simulink model "CommSysSimulink_Project2"  (R2024b)
settings: Solver=VariableStepAuto  StartTime=0.0  StopTime=inf  RelTol=1e-3
model workspace (MAT data in the model file):
  Data_Aided_Synchronisation = Simulink.Parameter
  Data_Aided_Synchronisation.Value = 0
  Data_Aided_Synchronisation.Complexity = 'real'
  Data_Aided_Synchronisation.Dimensions = [1 1]
  Data_Aided_Synchronisation.DataType = 'auto'
  Frequency_Locked_Loop = Simulink.Parameter
  Frequency_Locked_Loop.Value = 0
  Frequency_Locked_Loop.Complexity = 'real'
  Frequency_Locked_Loop.Dimensions = [1 1]
  Frequency_Locked_Loop.DataType = 'auto'
  Phase_Locked_Loop = Simulink.Parameter
  Phase_Locked_Loop.Value = 0
  Phase_Locked_Loop.Complexity = 'real'
  Phase_Locked_Loop.Dimensions = [1 1]
  Phase_Locked_Loop.DataType = 'auto'
  Symbol_Synchronisation = Simulink.Parameter
  Symbol_Synchronisation.Value = 0
  Symbol_Synchronisation.Complexity = 'real'
  Symbol_Synchronisation.Dimensions = [1 1]
  Symbol_Synchronisation.DataType = 'auto'
  Use_Costas_Loop = Simulink.Parameter
  Use_Costas_Loop.Value = 0
  Use_Costas_Loop.Complexity = 'real'
  Use_Costas_Loop.Dimensions = [1 1]
  Use_Costas_Loop.DataType = 'auto'
  iSNR = 1
  x = 0
undefined symbols (not defined in the file): alpha, fCRes, filterLenSymbols, modOrder, phaseOffsets, phaseOffsetSelector, samplesPerSymbol, SNR, symRate
libraries: commdigbbndpm3 x6, commsync2 x5, commrfcorlib x3, simulink x2, commfilt2 x2, commdigbbndam3 x2, commchan3 x1, commsink2 x1, commseqgen3 x1, commrandsrc3 x1, commrflib2 x1
settings Model: Creator=flora  LastModifiedBy=Sukhman

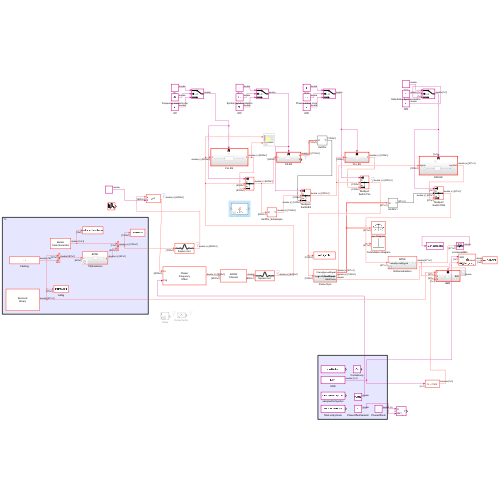
[thumbnail: Simulink's stored preview of the top-level diagram]
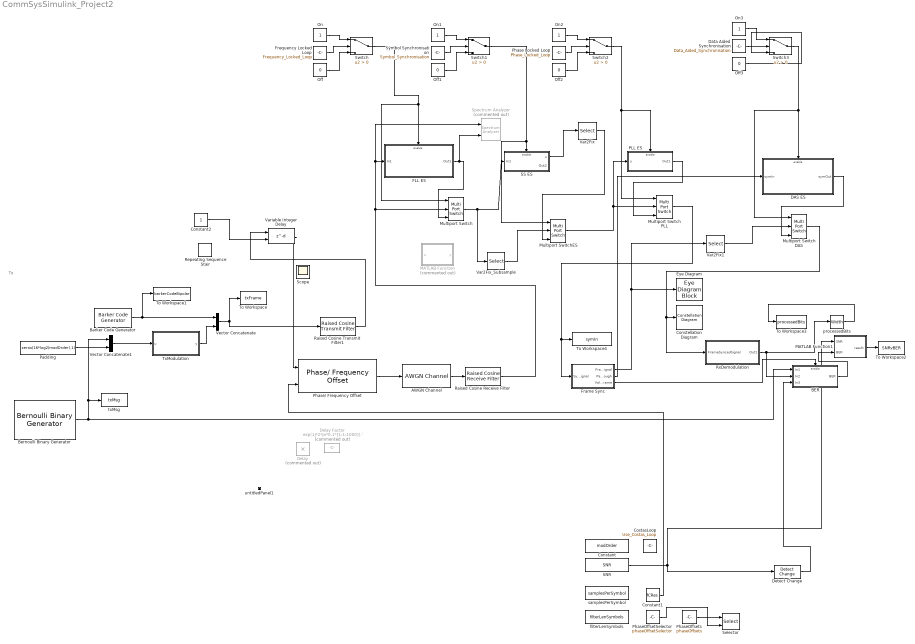
== system CommSysSimulink_Project2 ==
  note: Tx
  AWGN Channel : commchan3/AWGN Channel  LegacyMode=off  NoiseMethod="Signal to noise ratio  (Eb/No)"  noiseMode="Signal to noise ratio  (SNR)"  EbNo=SNR  EsNo=10  SNR=SNR  BitsPerSymbol=log2(modOrder)  SignalPower=1/samplesPerSymbol  SamplesPerSymbol=samplesPerSymbol  SymbolPeriod=1  VarianceSource=Parameter  Variance=SNR/2  RandomStream=Global stream  Seed=67  SimulateUsing=Interpreted execution
  BER : Subsystem  TreatAsAtomicUnit=on
  Barker Code Generator : commseqgen3/Barker Code Generator  Length=7  LengthSimulink=13  SampleTime=-1  SamplesPerFrame=13  OutputDataType=double  SimulateUsing=Interpreted execution
  Bernoulli Binary Generator : commrandsrc3/Bernoulli Binary Generator  ProbabilityOfZero=0.5  SeedSource=Auto  Seed=0  SampleTime=1/(symRate*log2(modOrder))  SamplesPerFrame="(symRate  - 13 -16) * log2(modOrder)"  OutputDataType=double  SimulateUsing=Interpreted execution
  Constant : Constant  Value=modOrder
  Constant1 : Constant  Value=fCRes
  Constant2 : Constant
  Constellation Diagram : ConstellationDiagram  WindowPosition=[527.000000,241.000000,653.000000,585.000000,]  Visible=on  ScopeFrameLocation=window  ReferenceConstellation=BPSK  XLimits=[-1.375,1.375]  YLimits=[-1.375,1.375]  MaximizeAxes=on
  CostasLoop : Constant  Value=Use_Costas_Loop
  DAS ES : Subsystem  TreatAsAtomicUnit=on
  Data Aided Synchronisation : Constant  Value=Data_Aided_Synchronisation  VectorParams1D=off
  Delay : Product  Commented=on  LockScale=on
  Delay Factor : Constant  Commented=on  Value=exp(1j*2*pi*0.1*[1:1:1000]).'  VectorParams1D=off  SampleTime=0.971  LockScale=on
  Detect Change : simulink/Logic and Bit Operations/Detect Change  vinit=0  OutDataTypeStr=boolean
  Eye Diagram : EyeDiagramBlock  WindowPosition=[302.000000,4.000000,1167.000000,855.000000,]  Visible=on  ScopeFrameLocation=window
  FLL ES : Subsystem  TreatAsAtomicUnit=on
  Frame Sync : Subsystem
  Frequency Locked Loop : Constant  Value=Frequency_Locked_Loop
  MATLAB Function : MATLAB Function  Commented=on  TreatAsAtomicUnit=on
  MATLAB Function1 : MATLAB Function  TreatAsAtomicUnit=on
  Multiport Switch : MultiPortSwitch  DataPortOrder=Zero-based contiguous  Inputs=2  zeroidx=on  SaturateOnIntegerOverflow=off  InputSameDT=off
  Multiport Switch DAS : MultiPortSwitch  DataPortOrder=Zero-based contiguous  Inputs=2  zeroidx=on  SaturateOnIntegerOverflow=off  InputSameDT=off
  Multiport Switch PLL : MultiPortSwitch  DataPortOrder=Zero-based contiguous  Inputs=2  zeroidx=on  SaturateOnIntegerOverflow=off  InputSameDT=off
  Multiport SwitchES : MultiPortSwitch  DataPortOrder=Zero-based contiguous  Inputs=2  zeroidx=on  SaturateOnIntegerOverflow=off  InputSameDT=off
  Off{,1..3} (4 alike) : Constant  Value=0
  On{,1..3} (4 alike) : Constant
  PLL ES : Subsystem  TreatAsAtomicUnit=on
  Padding : Constant  Value=zeros(16*log2(modOrder),1)  SampleTime=-1
  Phase Locked Loop : Constant  Value=Phase_Locked_Loop
  Phase/ Frequency Offset : commrflib2/Phase// Frequency Offset  phaseOffset=rad2deg(phaseOffsets(phaseOffsetSelector))  freqPort=on  freqOffset=100
      settings: LibrarySourceBlock=|
      | commrfcorlib/Phase//
      | Frequency
      | Offset
  PhaseOffsetSelector : Constant  Value=phaseOffsetSelector
  PhaseOffsets : Constant  Value=phaseOffsets
  Raised Cosine Receive Filter : commfilt2/Raised Cosine Receive Filter  filtType=Square root  R=alpha  filtSpan=filterLenSymbols  N=samplesPerSymbol  downFactor=1  downOffset=0  filterGain=1  InputProcessing=Columns as channels (frame based)  RateOptions=Enforce single-rate processing  framing=Mute  checkCoeff=on  variableName=rcRxFilt  currentFiltSpan=10  D=5  inputOffset=0  sampMode=Mute  saveAsFlag=0  rateMode=Downsampling  checkGain=Normalized  launchFVT=on  roundingMode=Floor  overflowMode=off  coeffDataTypeStr=Inherit: Same word length as input  coeffMin=[]  coeffMax=[]  coeffLastDataTypeStr=Inherit: Same word length as input  accumDataTypeStr=Inherit: Same as product output  accumLastDataTypeStr=Inherit: Same as product output  outputDataTypeStr=Inherit: Same as accumulator  outputMin=[]  outputMax=[]  outputLastDataTypeStr=Inherit: Same as accumulator
  Raised Cosine Transmit Filter1 : commfilt2/Raised Cosine Transmit Filter  filtType=Square root  R=alpha  filtSpan=filterLenSymbols  N=samplesPerSymbol  filterGain=1  InputProcessing=Columns as channels (frame based)  RateOptions=Enforce single-rate processing  framing=Mute  checkCoeff=on  variableName=rcTxFilt  checkGain=Normalized  sampMode=Mute  saveAsFlag=0  currentFiltSpan=10  D=(10)/2  launchFVT=on  roundingMode=Floor  overflowMode=off  coeffDataTypeStr=Inherit: Same word length as input  coeffMin=[]  coeffMax=[]  coeffLastDataTypeStr=Inherit: Same word length as input  outputDataTypeStr=Inherit: Same as accumulator  outputMin=[]  outputMax=[]  outputLastDataTypeStr=Inherit: Same as accumulator
  Repeating Sequence Stair : simulink/Sources/Repeating Sequence Stair  OutValues=[3 1 4 2 1].'  tsamp=-1  OutMin=[]  OutMax=[]  OutDataTypeStr=double  OutputDataTypeScalingMode=double  OutDataType=fixdt(0,8)  ConRadixGroup=Best Precision: Vector-wise  OutScaling=2^-12
      settings: LibrarySourceBlock=|
      | hdlsllib/Sources/Repeating
      | Sequence
      | Stair
  RxDemodulation : Subsystem  Variant=on
  SNR : Constant  Value=SNR  VectorParams1D=off
  SS ES : Subsystem  TreatAsAtomicUnit=on
  Selector : Selector  InputPortWidth=5  IndexOptions=Index vector (port)  Indices=[1 3]  OutputSizes=1
  Spectrum Analyzer : SpectrumAnalyzer  Commented=on  NumInputPorts=2  WindowPosition=[-1976.000000,107.000000,1455.000000,953.000000,]  Visible=on  ScopeFrameLocation=window  ViewType=Spectrum and spectrogram  PlotAsTwoSidedSpectrum=off  Span=399999.99999999994  StartFrequency=-199999.99999999997  StopFrequency=199999.99999999997  YLimits=[-112.84937781743083,24.09936467256917]  ColorLimits=[-112.30807844,24.64066405]  ExpandToolstrip=on
  Switch{,1..3} (4 alike) : Switch  Criteria=u2 > Threshold  SaturateOnIntegerOverflow=off  InputSameDT=off
  Symbol Synchronisation : Constant  Value=Symbol_Synchronisation
  To Workspace : ToWorkspace  VariableName=txFrame  SampleTime=-1
      settings: Save2DSignal=2-D array (concatenate along first dimension)
  To Workspace1 : ToWorkspace  VariableName=barkerCodeBipolar  SampleTime=-1
      settings: Save2DSignal=2-D array (concatenate along first dimension)
  To Workspace2 : ToWorkspace  VariableName=SNRvBER  SampleTime=-1
  To Workspace3 : ToWorkspace  VariableName=processedBits  SaveFormat=Timeseries  SampleTime=-1
  To Workspace4 : ToWorkspace  VariableName=symIn  SampleTime=-1
  TxModulation : Subsystem  Variant=on
  Var2Fix : Selector  InputPortWidth=symRate*1.1  IndexOptions=Starting index (dialog)  Indices=1  OutputSizes=symRate
  Var2Fix1 : Selector  InputPortWidth=symRate-13-16  IndexOptions=Starting index (dialog)  Indices=1  OutputSizes=symRate-13-16
  Var2Fix_Subsample : Selector  InputPortWidth=symRate*samplesPerSymbol  IndexOptions=Index vector (dialog)  Indices=[1: samplesPerSymbol : symRate*samplesPerSymbol]  OutputSizes=symRate*samplesPerSymbol
  Variable Integer Delay : Delay  DelayLengthSource=Input port  InputProcessing=Columns as channels (frame based)
      settings: InputPortMap=u0,p1
  Vector Concatenate : Concatenate
  Vector Concatenate1 : Concatenate
  filterLenSymbols : Constant  Value=filterLenSymbols
  processedBits : Width
  samplesPerSymbol : Constant  Value=samplesPerSymbol
  txMsg : ToWorkspace  VariableName=txMsg  SampleTime=-1
      settings: Save2DSignal=2-D array (concatenate along first dimension)
  untitledPanel1 : Subsystem  Tag=HiddenForWebPanel  IsWebBlockPanel=on
  Scope : Scope
  wires:
  BER/1(BER) -> MATLAB Function1/2(BER)
  processedBits/1 -> To Workspace3/1
  Detect Change/1 -> BER/3(In3)
  Frame Sync/1(FrameSyncedSignal) -> Var2Fix1/1, Eye Diagram/1
  AWGN Channel/1 -> Raised Cosine Receive Filter/1
  MATLAB Function1/1(result) -> To Workspace2/1
  RxDemodulation/1(Out1) -> processedBits/1, BER/2(In2)
  SNR/1 -> MATLAB Function1/1(SNR), Detect Change/1
  Frame Sync/3(ValidFrame) -> BER/Enable
  Bernoulli Binary Generator/1 -> txMsg/1, Vector Concatenate1/1, BER/1(In1)
  Barker Code Generator/1 -> Vector Concatenate/1, To Workspace1/1
  Vector Concatenate1/1 -> TxModulation/1(u)
  TxModulation/1(y) -> Vector Concatenate/2
  Padding/1 -> Vector Concatenate1/2
  Vector Concatenate/1 -> To Workspace/1, Raised Cosine Transmit Filter1/1
  Phase/ Frequency Offset/1 -> AWGN Channel/1
  PhaseOffsets/1 -> Selector/1
  PhaseOffsetSelector/1 -> Selector/2
  Constant1/1 -> Phase/ Frequency Offset/2
  On/1 -> Switch/1
  Off/1 -> Switch/3
  Frequency Locked Loop/1 -> Switch/2
  Switch/1 -> Multiport Switch/1, FLL ES/Enable
  Symbol Synchronisation/1 -> Switch1/2
  On1/1 -> Switch1/1
  Off1/1 -> Switch1/3
  Phase Locked Loop/1 -> Switch2/2
  Off2/1 -> Switch2/3
  On2/1 -> Switch2/1
  Switch1/1 -> Multiport SwitchES/1, SS ES/Enable
  Raised Cosine Receive Filter/1 -> Spectrum Analyzer/1, FLL ES/1(In1), Multiport Switch/2
  FLL ES/1(Out1) -> Spectrum Analyzer/2, Multiport Switch/3
  Multiport Switch/1 -> SS ES/1(In1), Var2Fix_Subsample/1
  Switch2/1 -> Multiport Switch PLL/1, PLL ES/Enable
  SS ES/1(u) -> Var2Fix/1
  PLL ES/1(Out1) -> Multiport Switch PLL/3
  Multiport Switch PLL/1 -> Frame Sync/1(SymbolSyncedSignal), To Workspace4/1
  Var2Fix/1 -> Multiport SwitchES/3
  Multiport SwitchES/1 -> PLL ES/1(u), Multiport Switch PLL/2
  Var2Fix_Subsample/1 -> Multiport SwitchES/2
  Raised Cosine Transmit Filter1/1 -> Variable Integer Delay/1
  Off3/1 -> Switch3/3
  Data Aided Synchronisation/1 -> Switch3/2
  On3/1 -> Switch3/1
  Switch3/1 -> Multiport Switch DAS/1, DAS ES/Enable
  DAS ES/1(symOut) -> Multiport Switch DAS/3
  Frame Sync/2(Passthrough) -> DAS ES/1(symIn)
  Multiport Switch DAS/1 -> RxDemodulation/1(FrameSyncedSignal), Constellation Diagram/1
  Var2Fix1/1 -> Multiport Switch DAS/2
  Constant2/1 -> Variable Integer Delay/2
  Variable Integer Delay/1 -> Phase/ Frequency Offset/1

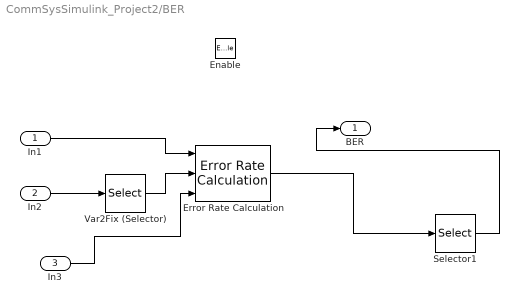
== system CommSysSimulink_Project2/BER ==
  In1 : Inport
  In2 : Inport  Port=2
  In3 : Inport  Port=3
  Enable : EnablePort  PropagateVarSize=During execution
  Error Rate Calculation : commsink2/Error Rate Calculation  N=0  st_delay=0  cp_mode=Entire frame  subframe=[]  PMode=Port  WsName=ErrorVec  RsMode2=on  stop=off  numErr=100  maxBits=1e6
      settings: LibrarySourceBlock=|
      | commhdlsink/Error Rate
      | Calculation
  Selector1 : Selector  InputPortWidth=3  IndexOptions=Index vector (dialog)  Indices=1  OutputSizes=1
  Var2Fix (Selector) : Selector  IndexOptions=Starting index (dialog)  Indices=1  OutputSizes="(symRate  - 13 -16) * log2(modOrder)"
  BER : Outport
  wires:
  In1/1 -> Error Rate Calculation/1
  Var2Fix (Selector)/1 -> Error Rate Calculation/2
  Error Rate Calculation/1 -> Selector1/1
  Selector1/1 -> BER/1
  In2/1 -> Var2Fix (Selector)/1
  In3/1 -> Error Rate Calculation/3

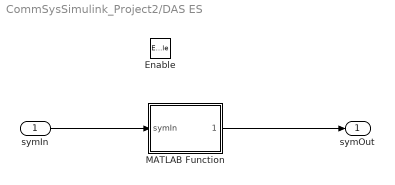
== system CommSysSimulink_Project2/DAS ES ==
  symIn : Inport
  Enable : EnablePort
  MATLAB Function : MATLAB Function  TreatAsAtomicUnit=on
  symOut : Outport
  wires:
  symIn/1 -> MATLAB Function/1(symIn)
  MATLAB Function/1(symOut) -> symOut/1

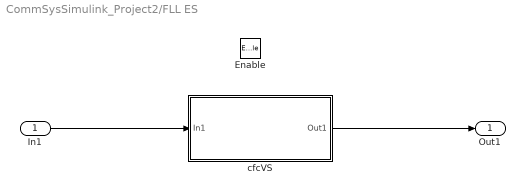
== system CommSysSimulink_Project2/FLL ES ==
  In1 : Inport
      settings: SignalType=complex
  Enable : EnablePort
  cfcVS : Subsystem  Variant=on
  Out1 : Outport
  wires:
  cfcVS/1(Out1) -> Out1/1
  In1/1 -> cfcVS/1(In1)

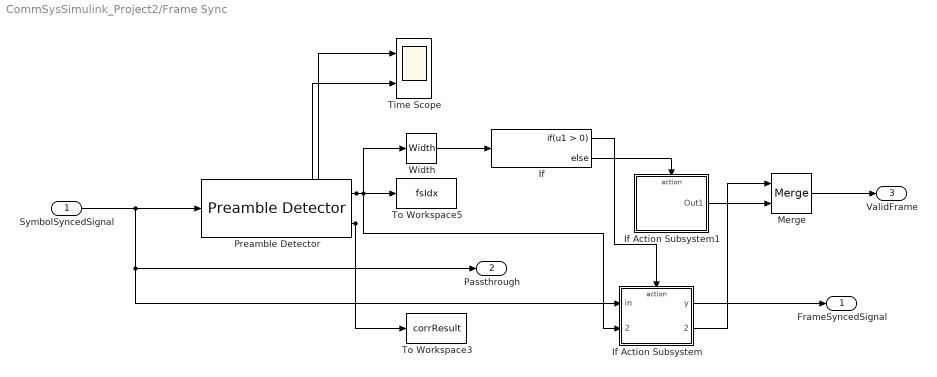
== system CommSysSimulink_Project2/Frame Sync ==
  SymbolSyncedSignal : Inport
  If : If
  If Action Subsystem : Subsystem  TreatAsAtomicUnit=on
  If Action Subsystem1 : Subsystem  TreatAsAtomicUnit=on
  Merge : Merge
  Preamble Detector : commsync2/Preamble Detector  Input=Symbol  Preamble=[-1;-1;-1;-1;-1;1;1;-1;-1;1;-1;1;-1]  Threshold=5  DetectionMetricOutput=on  Detections=First  SimulateUsing=Interpreted execution
  Time Scope : Scope  NumInputPorts=2
  To Workspace3 : ToWorkspace  VariableName=corrResult  SaveFormat=Timeseries  SampleTime=-1
      settings: Save2DSignal=2-D array (concatenate along first dimension)
  To Workspace5 : ToWorkspace  VariableName=fsIdx  SaveFormat=Structure  SampleTime=-1
  Width : Width
  FrameSyncedSignal : Outport
  Passthrough : Outport  Port=2
  ValidFrame : Outport  Port=3
  wires:
  If Action Subsystem/1(y) -> FrameSyncedSignal/1
  Merge/1 -> ValidFrame/1
  Width/1 -> If/1
  Preamble Detector/2 -> To Workspace3/1, Time Scope/2
  If/1 -> If Action Subsystem/Action
  Preamble Detector/1 -> Time Scope/1, If Action Subsystem/2(peakIdx), To Workspace5/1, Width/1
  If Action Subsystem1/1(Out1) -> Merge/2
  If/2 -> If Action Subsystem1/Action
  SymbolSyncedSignal/1 -> Preamble Detector/1, Passthrough/1, If Action Subsystem/1(in)
  If Action Subsystem/2(ValidFrame) -> Merge/1

== system CommSysSimulink_Project2/PLL ES ==
  u : Inport
  Enable : EnablePort  PropagateVarSize=During execution
  Variant Subsystem : Subsystem  Variant=on
  Out1 : Outport
  wires:
  u/1 -> Variant Subsystem/1(u)
  Variant Subsystem/1(y) -> Out1/1

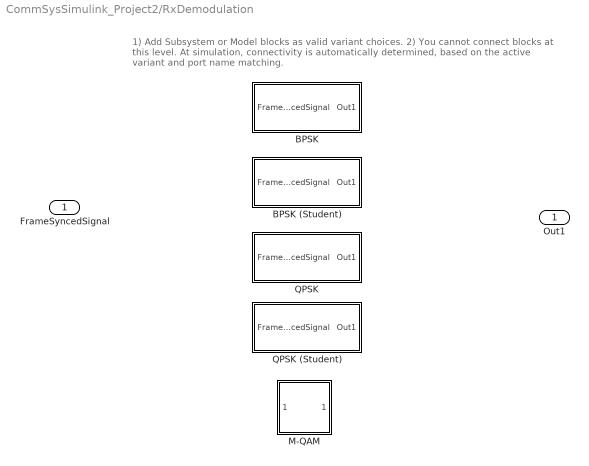
== system CommSysSimulink_Project2/RxDemodulation ==
  note: 1) Add Subsystem or Model blocks as valid variant choices.
      | 2) You cannot connect blocks at this level. At simulation, connectivity is automatically
      | determined, based on the active variant and port name matching.
  FrameSyncedSignal : Inport
  BPSK : Subsystem  VariantControl="modScheme==\"BPSK\""
  BPSK (Student) : Subsystem  VariantControl="modScheme==\"BPSK (Student)\""
  M-QAM : Subsystem  VariantControl="modScheme==\"M-QAM\""
  QPSK : Subsystem  VariantControl="modScheme==\"QPSK\""
  QPSK (Student) : Subsystem  VariantControl="modScheme==\"QPSK (Student)\""
  Out1 : Outport

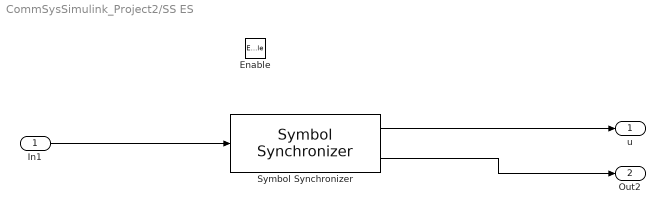
== system CommSysSimulink_Project2/SS ES ==
  In1 : Inport
  Enable : EnablePort  PropagateVarSize=During execution
  Symbol Synchronizer : commsync2/Symbol Synchronizer  Modulation=PAM/PSK/QAM  TimingErrorDetector=Zero-Crossing (decision-directed)  SamplesPerSymbol=samplesPerSymbol  DampingFactor=1  NormalizedLoopBandwidth=0.01  DetectorGain=2.7  TimingErrorOutputPort=on  SimulateUsing=Code generation
  u : Outport
      settings: SignalType=complex
  Out2 : Outport  Port=2
  wires:
  In1/1 -> Symbol Synchronizer/1
  Symbol Synchronizer/1 -> u/1
  Symbol Synchronizer/2 -> Out2/1

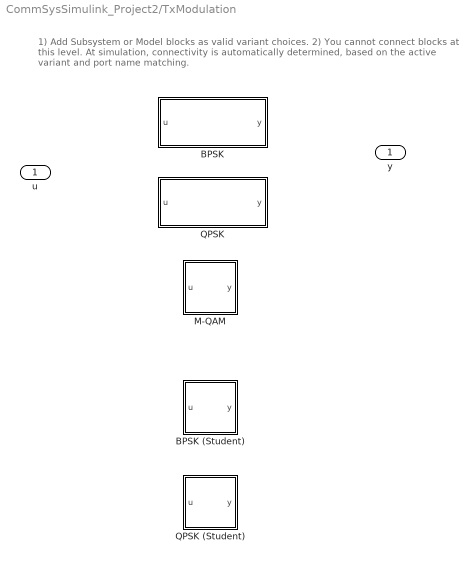
== system CommSysSimulink_Project2/TxModulation ==
  note: 1) Add Subsystem or Model blocks as valid variant choices.
      | 2) You cannot connect blocks at this level. At simulation, connectivity is automatically
      | determined, based on the active variant and port name matching.
  u : Inport
  BPSK : Subsystem  VariantControl="modScheme==\"BPSK\""
  BPSK (Student) : Subsystem  VariantControl="modScheme==\"BPSK (Student)\""
  M-QAM : Subsystem  VariantControl="modScheme==\"M-QAM\""
  QPSK : Subsystem  VariantControl="modScheme==\"QPSK\""
  QPSK (Student) : Subsystem  VariantControl="modScheme==\"QPSK (Student)\""
  y : Outport

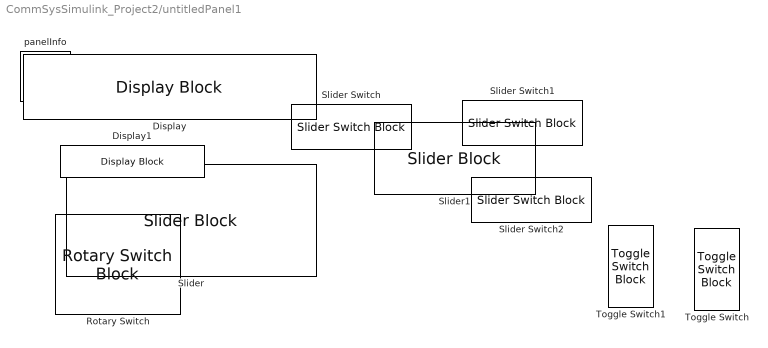
== system CommSysSimulink_Project2/untitledPanel1 ==
  Display : DisplayBlock  Tag=HiddenForWebPanel  PanelInfo="{\"height\":25,\"left\":685,\"panelId\":\"panelId-f31e1c61-8a53-45bb-afd0-f88e0f139d22\",\"top\":114,\"type\":\"panelChild\",\"version\":\"2019b\",\"width\":131,\"zIndex\":1500002}"  LabelPosition=Hide  Transparency=1
  Display1 : DisplayBlock  Tag=HiddenForWebPanel  PanelInfo="{\"height\":30,\"left\":680,\"panelId\":\"panelId-f31e1c61-8a53-45bb-afd0-f88e0f139d22\",\"top\":36,\"type\":\"panelChild\",\"version\":\"2019b\",\"width\":135,\"zIndex\":1500008}"  LabelPosition=Hide  Transparency=1
  Rotary Switch : RotarySwitchBlock  Tag=HiddenForWebPanel  PanelInfo="{\"height\":100,\"left\":271,\"panelId\":\"panelId-f31e1c61-8a53-45bb-afd0-f88e0f139d22\",\"top\":38,\"type\":\"panelChild\",\"version\":\"2019b\",\"width\":125,\"zIndex\":1500010}"  LabelPosition=Hide
      settings: Values={{'0', 'pi/8', 'pi/4', 'pi/2', 'pi'}, [1 2 3 4 5]}
  Slider : SliderBlock  Tag=HiddenForWebPanel  PanelInfo="{\"height\":88,\"left\":43,\"panelId\":\"panelId-f31e1c61-8a53-45bb-afd0-f88e0f139d22\",\"top\":53,\"type\":\"panelChild\",\"version\":\"2019b\",\"width\":191,\"zIndex\":1500006}"  ScaleMin=-30  ScaleMax=30
  Slider Switch : SliderSwitchBlock  Tag=HiddenForWebPanel  PanelInfo="{\"height\":45,\"left\":65,\"panelId\":\"panelId-f31e1c61-8a53-45bb-afd0-f88e0f139d22\",\"top\":226,\"type\":\"panelChild\",\"version\":\"2019b\",\"width\":120,\"zIndex\":1500014}"
      settings: Values={{'Off', 'On'}, [0 1]}
  Slider Switch1 : SliderSwitchBlock  Tag=HiddenForWebPanel  PanelInfo="{\"height\":45,\"left\":407,\"panelId\":\"panelId-f31e1c61-8a53-45bb-afd0-f88e0f139d22\",\"top\":225,\"type\":\"panelChild\",\"version\":\"2019b\",\"width\":120,\"zIndex\":1500016}"
      settings: Values={{'Off', 'On'}, [0 1]}
  Slider Switch2 : SliderSwitchBlock  Tag=HiddenForWebPanel  PanelInfo="{\"height\":45,\"left\":235,\"panelId\":\"panelId-f31e1c61-8a53-45bb-afd0-f88e0f139d22\",\"top\":225,\"type\":\"panelChild\",\"version\":\"2019b\",\"width\":120,\"zIndex\":1500018}"
      settings: Values={{'Off', 'On'}, [0 1]}
  Slider1 : SliderBlock  Tag=HiddenForWebPanel  PanelInfo="{\"height\":72,\"left\":420,\"panelId\":\"panelId-f31e1c61-8a53-45bb-afd0-f88e0f139d22\",\"top\":62,\"type\":\"panelChild\",\"version\":\"2019b\",\"width\":161,\"zIndex\":1500022}"  LabelPosition=Hide
  Toggle Switch : ToggleSwitchBlock  Tag=HiddenForWebPanel  PanelInfo="{\"height\":104,\"left\":706,\"panelId\":\"panelId-f31e1c61-8a53-45bb-afd0-f88e0f139d22\",\"top\":182,\"type\":\"panelChild\",\"version\":\"2019b\",\"width\":79,\"zIndex\":1500020}"  LabelPosition=Hide
      settings: Values={{'Off', 'On'}, [0 1]}
  Toggle Switch1 : ToggleSwitchBlock  Tag=HiddenForWebPanel  PanelInfo="{\"height\":106,\"left\":576,\"panelId\":\"panelId-f31e1c61-8a53-45bb-afd0-f88e0f139d22\",\"top\":177,\"type\":\"panelChild\",\"version\":\"2019b\",\"width\":86,\"zIndex\":1500024}"  LabelPosition=Hide
      settings: Values={{'Off', 'On'}, [0 1]}
  panelInfo : PanelWebBlock  Tag=HiddenForWebPanel  PanelInfo="{\"compacted\":false,\"height\":321,\"isActiveTab\":true,\"labels\":{\"label1660874785\":{\"deleted\":false,\"left\":288,\"settings\":{\"backgroundColor\":\"rgba(0, 0, 0, 0)\",\"bold\":false,\"font\":\"Arial\",\"fontColor\":\"black\",\"fontSize\":0.9,\"italicized\":false,\"underlined\":false},\"text\":\"LO Phase Offset\",\"top\":15},\"label2052262155\":{\"deleted\":false,\"id\":\"label2052262155\",\"left\":43,\"settings\":{\"backgroundColor\":\"rgba(0, 0, 0, 0)\",\"bold\":false,\"font\":\"Arial\",\"fontColor\":\"black\",\"fontSize\":0.84,\"italicized\":false,\"underlined\":false},\"text\":\"SNR (dB)\",\"top\":31},\"label3800272950\":{\"deleted\":false,\"id\":\"label3800272950\",\"left\":678,\"settings\":{\"backgroundColor\":\"rgba(0, 0, 0, 0)\",\"bold\":false,\"font\":\"Arial\",\"fontColor\":\"black\",\"fontSize\":0.84,\"italicized\":false,\"underlined\":false},\"text\":\"Processed Bits\",\"top\":91},\"label4504685010\":{\"deleted\":false,\"left\":570,\"settings\":{\"backgroundColor\":\"rgba(0, 0, 0, 0)\",\"bold\":false,\"font\":\"Arial\",\"fontColor\":\"black\",\"fontSize\":0.9,\"italicized\":false,\"underlined\":false},\"text\":\"Data-aided sync\",\"top\":287},\"label4915582058\":{\"deleted\":false,\"left\":440,\"settings\":{\"backgroundColor\":\"rgba(0, 0, 0, 0)\",\"bold\":false,\"font\":\"Arial\",\"fontColor\":\"black\",\"fontSize\":0.9,\"italicized\":false,\"underlined\":false},\"text\":\"LO Frequency Offset\",\"top\":40},\"label7051701793\":{\"deleted\":false,\"id\":\"label7051701793\",\"left\":676,\"settings\":{\"backgroundColor\":\"rgba(0, 0, 0, 0)\",\"bold\":false,\"font\":\"Arial\",\"fontColor\":\"black\",\"fontSize\":0.84,\"italicized\":false,\"underlined\":false},\"text\":\"BER\",\"top\":14},\"label8369097741\":{\"deleted\":false,\"left\":694,\"settings\":{\"backgroundColor\":\"rgba(0, 0, 0, 0)\",\"bold\":false,\"font\":\"Arial\",\"fontColor\":\"black\",\"fontSize\":0.9,\"italicized\":false,\"underlined\":false},\"text\":\"Use Costas Loop\",\"top\":289}},\"left\":160,\"name\":\"Communication System Dashboard\",\"panelId\":\"panelId-f31e1c61-8a53-45bb-afd0-f88e0f139d22\",\"popoutData\":{\"height\":688,\"left\":-14,\"maximized\":false,\"top\":316,\"width\":829},\"popoutMode\":\"window\",\"tabIndex\":0,\"tabbedSetId\":\"tabbedSet4545170372\",\"top\":32,\"type\":\"panel\",\"version\":\"2019b\",\"visible\":true,\"width\":855,\"zIndex\":1500002}"  PanelSnapshot=<binary blob, 30424 chars, not shown>

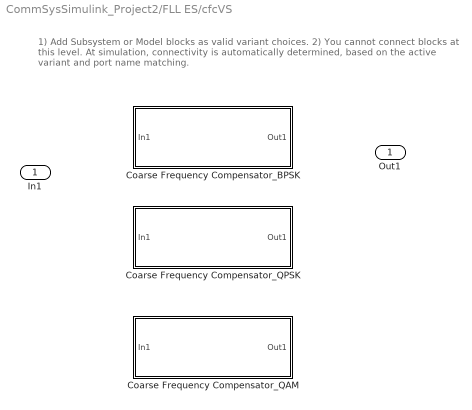
== system CommSysSimulink_Project2/FLL ES/cfcVS ==
  note: 1) Add Subsystem or Model blocks as valid variant choices.
      | 2) You cannot connect blocks at this level. At simulation, connectivity is automatically
      | determined, based on the active variant and port name matching.
  In1 : Inport
  Coarse Frequency Compensator_BPSK : Subsystem  VariantControl="modScheme == \"BPSK\""
  Coarse Frequency Compensator_QAM : Subsystem  VariantControl="modScheme == \"QAM\""
  Coarse Frequency Compensator_QPSK : Subsystem  VariantControl="modScheme == \"QPSK\""
  Out1 : Outport

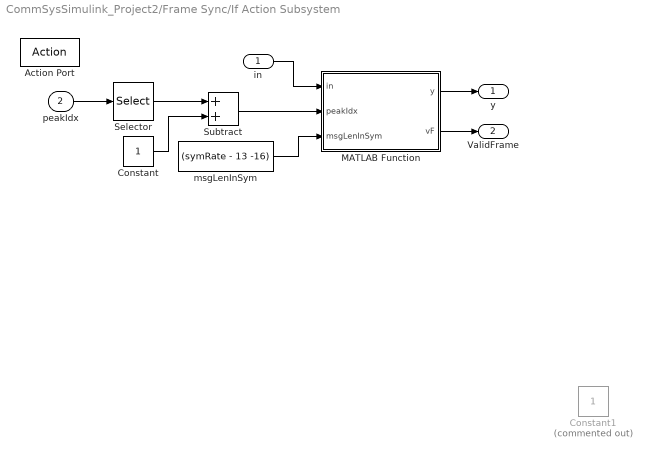
== system CommSysSimulink_Project2/Frame Sync/If Action Subsystem ==
  in : Inport
  peakIdx : Inport  Port=2
  Action Port : ActionPort  PropagateVarSize=During execution  ActionPortLabel=if(u1 > 0)
  Constant : Constant
  Constant1 : Constant  Commented=on
  MATLAB Function : MATLAB Function  TreatAsAtomicUnit=on
  Selector : Selector  InputPortWidth=1  IndexOptions=Index vector (dialog)  Indices=1  OutputSizes=1
  Subtract : Sum
  msgLenInSym : Constant  Value="(symRate  - 13 -16)"
  y : Outport
  ValidFrame : Outport  Port=2
  wires:
  MATLAB Function/1(y) -> y/1
  msgLenInSym/1 -> MATLAB Function/3(msgLenInSym)
  Constant/1 -> Subtract/2
  Subtract/1 -> MATLAB Function/2(peakIdx)
  in/1 -> MATLAB Function/1(in)
  Selector/1 -> Subtract/1
  MATLAB Function/2(vF) -> ValidFrame/1
  peakIdx/1 -> Selector/1

== system CommSysSimulink_Project2/Frame Sync/If Action Subsystem1 ==
  Action Port : ActionPort  ActionPortLabel=else
  Constant : Constant  Value=0
  Out1 : Outport
  wires:
  Constant/1 -> Out1/1

== system CommSysSimulink_Project2/PLL ES/Variant Subsystem ==
  note: 1) Add Subsystem or Model blocks as valid variant choices.
      | 2) You cannot connect blocks at this level. At simulation, connectivity is automatically
      | determined, based on the active variant and port name matching.
  u : Inport
  Costas Loop : Subsystem  VariantControl=Use_Costas_Loop == 1
  Default : Subsystem  VariantControl=Use_Costas_Loop == 0
  y : Outport

== system CommSysSimulink_Project2/RxDemodulation/BPSK ==
  FrameSyncedSignal : Inport
  BPSK Demodulator Baseband : commdigbbndpm3/BPSK Demodulator Baseband  DecType=Hard decision  VarSource=Dialog  Variance=1  Ph=0  outDtype=Inherit via internal rule  derotateFactorWordLen=16  derotateFactorDataTypeStr=Inherit: Same word length as input  derotateFactorLastDataTypeStr=Inherit: Same word length as input
  Out1 : Outport
  wires:
  FrameSyncedSignal/1 -> BPSK Demodulator Baseband/1
  BPSK Demodulator Baseband/1 -> Out1/1

== system CommSysSimulink_Project2/RxDemodulation/BPSK (Student) ==
  FrameSyncedSignal : Inport
  BPSK Demodulator Baseband : commdigbbndpm3/BPSK Demodulator Baseband  DecType=Hard decision  VarSource=Dialog  Variance=1  Ph=0  outDtype=Inherit via internal rule  derotateFactorWordLen=16  derotateFactorDataTypeStr=Inherit: Same word length as input  derotateFactorLastDataTypeStr=Inherit: Same word length as input
  Out1 : Outport
  wires:
  FrameSyncedSignal/1 -> BPSK Demodulator Baseband/1
  BPSK Demodulator Baseband/1 -> Out1/1

== system CommSysSimulink_Project2/RxDemodulation/M-QAM ==
  FrameSyncedSignal : Inport
  Rectangular QAM Demodulator Baseband : commdigbbndam3/Rectangular QAM Demodulator Baseband  M=modOrder  OutType=Bit  DecType=Hard decision  VarSource=Dialog  Variance=1  Dec=Gray  Mapping=[0:15]  PowType=Peak Power  MinDist=2  AvgPow=1  PeakPow=1  Ph=0  outDtype1=Inherit via internal rule  outDtype2=Inherit via internal rule  derotateFactorWordLen=16  derotateFactorDataTypeStr=Inherit: Same word length as input  derotateFactorLastDataTypeStr=Inherit: Same word length as input  denormFactorWordLen=16  denormFactorDataTypeStr=Inherit: Same word length as input  denormFactorLastDataTypeStr=Inherit: Same word length as input  prodOutWordLen=32  prodOutOverflowMode=Wrap  prodOutRoundingMode=Floor  prodOutOvFlMode=off  prodOutOvFlModeLastStrValue=off  sumWordLen=32
  Out1 : Outport
  wires:
  FrameSyncedSignal/1 -> Rectangular QAM Demodulator Baseband/1
  Rectangular QAM Demodulator Baseband/1 -> Out1/1

== system CommSysSimulink_Project2/RxDemodulation/QPSK ==
  FrameSyncedSignal : Inport
  QPSK Demodulator Baseband : commdigbbndpm3/QPSK Demodulator Baseband  OutType=Bit  DecType=Hard decision  VarSource=Dialog  Variance=1  Dec=Gray  Ph=pi/4  outDtype1=Inherit via internal rule  outDtype2=Inherit via internal rule  derotateFactorWordLen=16  derotateFactorDataTypeStr=Inherit: Same word length as input  derotateFactorLastDataTypeStr=Inherit: Same word length as input
      settings: LibrarySourceBlock=|
      | commhdldigbbndpm/QPSK
      | Demodulator
      | Baseband
  Out1 : Outport
  wires:
  FrameSyncedSignal/1 -> QPSK Demodulator Baseband/1
  QPSK Demodulator Baseband/1 -> Out1/1

== system CommSysSimulink_Project2/RxDemodulation/QPSK (Student) ==
  FrameSyncedSignal : Inport
  QPSK Demodulator Baseband : commdigbbndpm3/QPSK Demodulator Baseband  OutType=Bit  DecType=Hard decision  VarSource=Dialog  Variance=1  Dec=Gray  Ph=pi/4  outDtype1=Inherit via internal rule  outDtype2=Inherit via internal rule  derotateFactorWordLen=16  derotateFactorDataTypeStr=Inherit: Same word length as input  derotateFactorLastDataTypeStr=Inherit: Same word length as input
      settings: LibrarySourceBlock=|
      | commhdldigbbndpm/QPSK
      | Demodulator
      | Baseband
  Out1 : Outport
  wires:
  FrameSyncedSignal/1 -> QPSK Demodulator Baseband/1
  QPSK Demodulator Baseband/1 -> Out1/1

== system CommSysSimulink_Project2/TxModulation/BPSK ==
  u : Inport
  BPSK Modulator Baseband : commdigbbndpm3/BPSK Modulator Baseband  Ph=0  outDtype=double  outWordLen=16  outUDDataType=sfix(16)  outFracLenMode=Best precision  outFracLen=15  outDataTypeStr=double  outLastDataTypeStr=double
  y : Outport
  wires:
  u/1 -> BPSK Modulator Baseband/1
  BPSK Modulator Baseband/1 -> y/1

== system CommSysSimulink_Project2/TxModulation/BPSK (Student) ==
  u : Inport
  MATLAB Function : MATLAB Function  TreatAsAtomicUnit=on
  y : Outport
  wires:
  u/1 -> MATLAB Function/1(u)
  MATLAB Function/1(y) -> y/1

== system CommSysSimulink_Project2/TxModulation/M-QAM ==
  u : Inport
  Rectangular QAM Modulator Baseband : commdigbbndam3/Rectangular QAM Modulator Baseband  M=modOrder  InType=Bit  Enc=Gray  Mapping=[0:15]  PowType=Peak Power  MinDist=2  AvgPow=1  PeakPow=1  Ph=0  outDtype=double  outWordLen=16  outUDDataType=sfix(16)  outFracLenMode=Best precision  outFracLen=15  outDataTypeStr=double  outLastDataTypeStr=double
  y : Outport
  wires:
  u/1 -> Rectangular QAM Modulator Baseband/1
  Rectangular QAM Modulator Baseband/1 -> y/1

== system CommSysSimulink_Project2/TxModulation/QPSK ==
  u : Inport
  QPSK Modulator Baseband : commdigbbndpm3/QPSK Modulator Baseband  InType=Bit  Enc=Gray  Ph=pi/4  outDtype=double  outWordLen=16  outUDDataType=sfix(16)  outFracLenMode=Best precision  outFracLen=15  outDataTypeStr=double  outLastDataTypeStr=double
      settings: LibrarySourceBlock=|
      | commhdldigbbndpm/QPSK
      | Modulator
      | Baseband
  y : Outport
  wires:
  u/1 -> QPSK Modulator Baseband/1
  QPSK Modulator Baseband/1 -> y/1

== system CommSysSimulink_Project2/TxModulation/QPSK (Student) ==
  u : Inport
  MATLAB Function : MATLAB Function  TreatAsAtomicUnit=on
  y : Outport
  wires:
  u/1 -> MATLAB Function/1(u)
  MATLAB Function/1(y) -> y/1

== system CommSysSimulink_Project2/FLL ES/cfcVS/Coarse Frequency Compensator_BPSK ==
  In1 : Inport
  Coarse Frequency Compensator : commrfcorlib/Coarse Frequency Compensator  Modulation=BPSK  Algorithm=FFT-based  FrequencyResolution=1  MaximumFrequencyOffset=5e3  SamplesPerSymbol=4  EstimatedFreqOffsetPort=off  SimulateUsing=Code generation
      settings: LibrarySourceBlock=|
      | commsync2/Coarse Frequency
      | Compensator
  Out1 : Outport
  wires:
  Coarse Frequency Compensator/1 -> Out1/1
  In1/1 -> Coarse Frequency Compensator/1

== system CommSysSimulink_Project2/FLL ES/cfcVS/Coarse Frequency Compensator_QAM ==
  In1 : Inport
  Coarse Frequency Compensator : commrfcorlib/Coarse Frequency Compensator  Modulation=QAM  Algorithm=FFT-based  FrequencyResolution=1  MaximumFrequencyOffset=5e3  SamplesPerSymbol=4  EstimatedFreqOffsetPort=off  SimulateUsing=Code generation
      settings: LibrarySourceBlock=|
      | commsync2/Coarse Frequency
      | Compensator
  Out1 : Outport
  wires:
  Coarse Frequency Compensator/1 -> Out1/1
  In1/1 -> Coarse Frequency Compensator/1

== system CommSysSimulink_Project2/FLL ES/cfcVS/Coarse Frequency Compensator_QPSK ==
  In1 : Inport
  Coarse Frequency Compensator : commrfcorlib/Coarse Frequency Compensator  Modulation=QPSK  Algorithm=FFT-based  FrequencyResolution=1  MaximumFrequencyOffset=5e3  SamplesPerSymbol=4  EstimatedFreqOffsetPort=off  SimulateUsing=Code generation
      settings: LibrarySourceBlock=|
      | commsync2/Coarse Frequency
      | Compensator
  Out1 : Outport
  wires:
  Coarse Frequency Compensator/1 -> Out1/1
  In1/1 -> Coarse Frequency Compensator/1

== system CommSysSimulink_Project2/PLL ES/Variant Subsystem/Costas Loop ==
  u : Inport
  MATLAB Function : MATLAB Function  TreatAsAtomicUnit=on
  y : Outport
  wires:
  u/1 -> MATLAB Function/1(symIn)
  MATLAB Function/1(symOut) -> y/1

== system CommSysSimulink_Project2/PLL ES/Variant Subsystem/Default ==
  u : Inport
  CarrierRecoveryModSchemeVS : Subsystem  Variant=on
  y : Outport
  wires:
  u/1 -> CarrierRecoveryModSchemeVS/1(u)
  CarrierRecoveryModSchemeVS/1(y) -> y/1

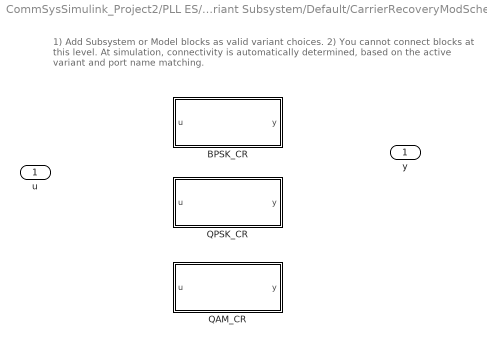
== system CommSysSimulink_Project2/PLL ES/Variant Subsystem/Default/CarrierRecoveryModSchemeVS ==
  note: 1) Add Subsystem or Model blocks as valid variant choices.
      | 2) You cannot connect blocks at this level. At simulation, connectivity is automatically
      | determined, based on the active variant and port name matching.
  u : Inport
  BPSK_CR : Subsystem  VariantControl="modScheme == \"BPSK\" || modScheme == \"BPSK (Student)\""
  QAM_CR : Subsystem  VariantControl="modScheme == \"QAM\""
  QPSK_CR : Subsystem  VariantControl="modScheme == \"QPSK\" || modScheme == \"QPSK (Student)\""
  y : Outport

== system CommSysSimulink_Project2/PLL ES/Variant Subsystem/Default/CarrierRecoveryModSchemeVS/BPSK_CR ==
  u : Inport
  PLL ES : commsync2/Carrier Synchronizer  Modulation=BPSK  ModulationPhaseOffset=Custom  CustomPhaseOffset=0  SamplesPerSymbol=1  DampingFactor=0.707  NormalizedLoopBandwidth=0.01  EstimatedPhaseErrorOutputPort=on  SimulateUsing=Code generation
  y : Outport
  wires:
  u/1 -> PLL ES/1
  PLL ES/1 -> y/1

== system CommSysSimulink_Project2/PLL ES/Variant Subsystem/Default/CarrierRecoveryModSchemeVS/QAM_CR ==
  u : Inport
  PLL ES : commsync2/Carrier Synchronizer  Modulation=QAM  ModulationPhaseOffset=Auto  CustomPhaseOffset=0  SamplesPerSymbol=1  DampingFactor=0.707  NormalizedLoopBandwidth=0.01  EstimatedPhaseErrorOutputPort=on  SimulateUsing=Code generation
  y : Outport
  wires:
  u/1 -> PLL ES/1
  PLL ES/1 -> y/1

== system CommSysSimulink_Project2/PLL ES/Variant Subsystem/Default/CarrierRecoveryModSchemeVS/QPSK_CR ==
  u : Inport
  PLL ES : commsync2/Carrier Synchronizer  Modulation=QPSK  ModulationPhaseOffset=Auto  CustomPhaseOffset=0  SamplesPerSymbol=1  DampingFactor=0.707  NormalizedLoopBandwidth=0.01  EstimatedPhaseErrorOutputPort=on  SimulateUsing=Code generation
  y : Outport
  wires:
  u/1 -> PLL ES/1
  PLL ES/1 -> y/1

== matlab function CommSysSimulink_Project2/Frame Sync/If Action Subsystem/MATLAB Function ==
  data: in input; y output size=[(symRate  - 13 -16) 1]; peakIdx input; msgLenInSym input; vF output
function [y,vF] = extractFrame(in,peakIdx, msgLenInSym)

    coder.varsize("y") % declares variables as variable-sized
   
    y = (0*0j) * zeros(msgLenInSym, 1);

    % Boundary check
    if (peakIdx + msgLenInSym - 1) > size(in, 1)
        vF = 0;
        return 
    end

    for i = 1: msgLenInSym
        y(i,1) = in(peakIdx  + (i-1));
    end

    vF = 1;
end

== matlab function CommSysSimulink_Project2/MATLAB Function ==
  data: u input; y output
function y = var2Fix(u)
    % Get the number of elements in the input array
    N = length(u);

    y = zeros(10000,1);

    

    
    % Create an array with values [1 2 ... N]
    y = 1:N;
end

== matlab function CommSysSimulink_Project2/TxModulation/BPSK (Student)/MATLAB Function ==
  data: u input; y output
function y = iBPSKmod(u)
% internal BPSKmod


coder.extrinsic("BPSKmod")
y = (0 +0i) * ones(size(u));

y = BPSKmod(u);

== matlab function CommSysSimulink_Project2/TxModulation/QPSK (Student)/MATLAB Function ==
  data: u input; y output
function y = iQPSKmod(u)
% internal BPSKmod


coder.extrinsic("QPSKmod")
y = (0 +0i) * ones(size(u,1)/2,1);  % Output is complex

y = QPSKmod(u);

== matlab function CommSysSimulink_Project2/MATLAB Function1 ==
  data: SNR input; result output; BER input
function result = snr_ber_array(SNR, BER)
    % Function to return a 2D array with the given SNR and BER values
    %
    % Inputs:
    %   SNR - Signal-to-Noise Ratio (scalar)
    %   BER - Bit Error Rate (scalar)
    %
    % Output:
    %   result - 2D array containing the SNR and BER values
    
    % Ensure the inputs are scalar
    if ~isscalar(SNR) || ~isscalar(BER)
        error('Both SNR and BER must be scalar values.');
    end
    
    % Create a 2D array with SNR and BER
    result = [SNR, BER];
end

== matlab function CommSysSimulink_Project2/PLL ES/Variant Subsystem/Costas Loop/MATLAB Function ==
  data: symIn input; symOut output
function symOut = iCostasLoop(symIn)

coder.extrinsic("costasLoop");

symOut = zeros(size(symIn)) * (0+0j);

symOut = costasLoop(symIn);

== matlab function CommSysSimulink_Project2/DAS ES/MATLAB Function ==
  data: symIn input; symOut output
function symOut = iDataAidedSync(symIn)

coder.extrinsic("dataAidedSync");

% Preamble is removed (+ padding is removed as well)
symOut = zeros(size(symIn,1)-13-16, size(symIn,2)) * (0+0j);


symOutDummy = dataAidedSync(symIn);

len = length(symOutDummy);

% Remove Padding (of length 16)
symOut = symOutDummy(1:987-16);


end
